simulink model "mdl_robot2"  (R2021b)
settings: Solver=VariableStepAuto  StartTime=0.0  StopTime=10.0  RelTol=1e-3
model workspace: external: MAT-File Robot_mdl_Workspace.mat (data not in the file)
libraries: SignalEditorBlockLib x1
settings Model: DataDictionary=Parent.sldd  EnableAccessToBaseWorkspace=off  Creator=hugo  LastModifiedBy=hugo
settings SolverCC: AlgebraicLoopSolver=TrustRegion
settings DataIOCC: ReturnWorkspaceOutputs=off
settings DebuggingCC: SFMachineParentedDataDiag=warning  ArithmeticOperatorsInVariantConditions=warning
settings ModelReferenceCC: ModelReferenceMinAlgLoopOccurrences=on
settings SFSimCC: SimUseLocalCustomCode=off  CustomCodeUndefinedFunction=UseInterfaceOnly
settings RTWCC: RTWUseLocalCustomCode=off

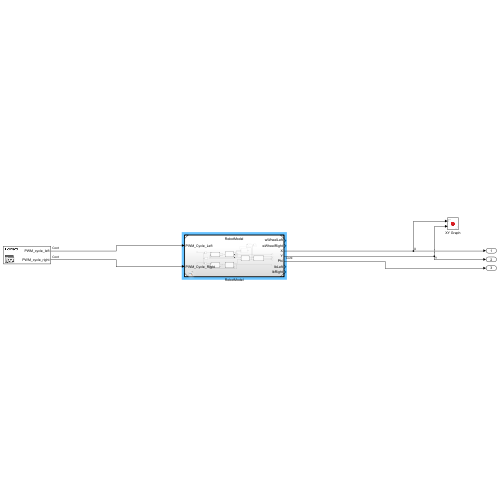
[thumbnail: Simulink's stored preview of the top-level diagram]
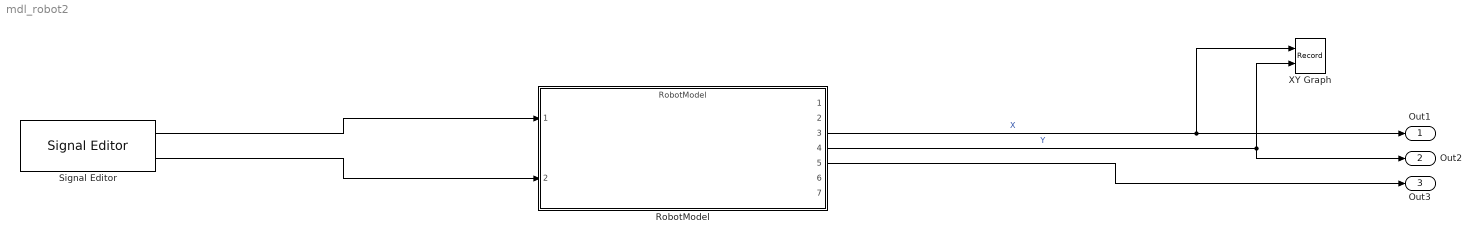
== system mdl_robot2 ==
  RobotModel : ModelReference  ModelNameDialog=RobotModel  SimulationMode=Normal  ModelReferenceVersion=1.55
  Signal Editor : SignalEditorBlockLib/Signal Editor  FileName=C:\Travail\EIRBOT\MMI\Asserv\Schema\Scenario\Scenario.mat  ActiveScenario=Forward  ActiveSignal=PWM_cycle_right  IsBus=off  OutputBusObjectStr=Bus: BusObject  SampleTime=0  ZeroCross=off  OutputAfterFinalValue=Setting to zero  Unit=inherit  PreserveSignalName=on
  XY Graph : Record  FileSettingsInternal="{\"entries\":[{\"content\":{\"excelSettings\":{\"content\":{},\"type\":\"Streamout.ExcelSettings\"}},\"type\":\"Streamout.FileSettingStorage\",\"uuid\":\"87c7be7d-2f54-4bd9-9e11-771c46b189eb\"}],\"packageUris\":[\"http://schema.mathworks.com/mf0/streamout_blocks/R2020a\"],\"version\":\"1.0\"}"  Layout=[1 1]  SignalsInternal="{\"entries\":[{\"content\":{\"signals\":[{\"content\":{\"blockPath\":[\"mdl_robot2/XY Graph\"],\"channel\":[],\"dimensions\":[1],\"domain\":\"mdl_robot2/XY Graph\",\"lineColor\":\"#a2142f\",\"plots\":[1],\"port\":1,\"sid\":[],\"signalID\":53,\"signalName\":\"XY Graph:1\"},\"type\":\"RecordBlkView.Signal\",\"uuid\":\"e80a43f2-82f5-4400-82bf-67c89005f6bf\"},{\"content\":{\"blockPath\":[\"mdl_robot2/XY Graph\"],\"channel\":[],\"dimensions\":[1],\"domain\":\"mdl_robot2/XY Graph\",\"lineColor\":\"#139fff\",\"plots\":[1],\"port\":2,\"sid\":[],\"signalID\":56,\"signalName\":\"XY Graph:2\"},\"type\":\"RecordBlkView.Signal\",\"uuid\":\"eb6c2693-9f07-40bf-b5e7-5ad4eaa929f6\"}]},\"type\":\"RecordBlkView.InputSignals\",\"uuid\":\"c987ee13-053d-4a13-a450-5733b6ad8903\"}],\"packageUris\":[\"http://schema.mathworks.com/mf0/streamout_blocks/R2020a\"],\"version\":\"1.0\"}"  VisualizationBindings="{\"xyplotplugin\":{\"info\":[{\"series\":[{\"bindingParametersList\":[{\"parameter\":\"X-Axis\",\"signalID\":53,\"signalName\":\"XY Graph:1\"},{\"parameter\":\"Y-Axis\",\"signalID\":56,\"signalName\":\"XY Graph:2\"}],\"seriesID\":57746}],\"subplotID\":1}]}}"  CompatibilityTag=XY  st=-1
  Out1 : Outport  VectorParamsAs1DForOutWhenUnconnected=off
  Out2 : Outport  Port=2  VectorParamsAs1DForOutWhenUnconnected=off
  Out3 : Outport  Port=3  VectorParamsAs1DForOutWhenUnconnected=off
  wires:
  Signal Editor/1 -> RobotModel/1
  Signal Editor/2 -> RobotModel/2
  RobotModel/5 -> Out3/1
  RobotModel/3 -> XY Graph/1, Out1/1  "X"
  RobotModel/4 -> Out2/1, XY Graph/2  "Y"
